simulink model "FloatShield_PID_Alternative"  (R2019a)
settings: Solver=FixedStepDiscrete  StartTime=0.0  StopTime=Inf  FixedStep=0.025  RelTol=1e-3
libraries: FloatLibrary x1, simulink x1
settings Model: SimulationMode=external  ExtModeTrigDuration=1  Creator=Peter  LastModifiedBy=Peter
settings OptimizationCC: EnhancedBackFolding=on  PassReuseOutputArgsAs=Individual arguments  MaxStackSize=64  OptimizeBlockOrder=speed  DifferentSizesBufferReuse=on  OptimizationCustomize=off
settings DebuggingCC: ParameterTunabilityLossMsg=error
settings HardwareCC: ProdBitPerInt=16  ProdBitPerPointer=16  ProdBitPerSizeT=16  ProdBitPerPtrDiffT=16  ProdLargestAtomicFloat=None  ProdWordSize=8  ProdHWDeviceType=Atmel->AVR
settings SFSimCC: MATLABDynamicMemAlloc=off
settings RTWCC: SystemTargetFile=ert.tlc  HardwareBoard=Arduino Uno  TLCOptions=-aInlineSetEventsForThisBaseRateFcn=TLC_FALSE -aSuppressMultiTaskScheduler=TLC_FALSE -aRateBasedStepFcn=1  TemplateMakefile=ert_default_tmf  GenerateReport=on  Toolchain=Arduino AVR  BuildConfiguration=Faster Runs  IncludeHyperlinkInReport=on  LaunchReport=on  GenerateTraceInfo=on  GenerateTraceReport=on  GenerateTraceReportSl=on  GenerateTraceReportSf=on  GenerateTraceReportEml=on
settings CodeAppCC: ForceParamTrailComments=on  IgnoreCustomStorageClasses=off  OperatorAnnotations=on  SimulinkDataObjDesc=on  SFDataObjDesc=on  InsertBlockDesc=on
settings ERTTargetCC: SupportContinuousTime=on  SupportVariableSizeSignals=on  ExtMode=on  ExtModeStaticAllocSize=250  ExtModeMexArgs='127.0.0.1' 0 17725

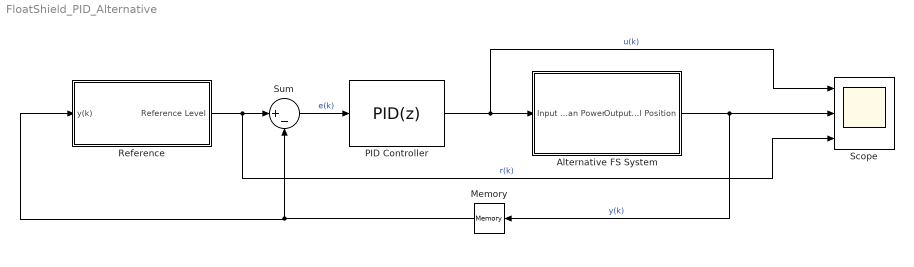
== system FloatShield_PID_Alternative ==
  Alternative FS System : Subsystem  mask{OutRadio=Percentage (%), Ncal=100, Ts=0.025}
      mask prompts: OutRadio "Output type"; Ncal "Calibration samples (-):"; Ts "Sampling period (s):"
      mask TypeOptions OutRadio: Percentage (%) | Altitude (mm)
      mask DialogControl DescGroupVar Prompt: FloatShield
      mask DialogControl DescTextVar Prompt: The block represents the FloatShield device. It accepts an input signal in the range of 0-100% that controls the fan power level and outputs ball position in form selected by the user. The block requires a sampling period and number of calibration samples out of which the extreme reading values will be computed using their mean value.
      mask Display: image('assets\FloatShield.svg');
  Memory : Memory  InheritSampleTime=on
  PID Controller : simulink/Continuous/PID Controller  Controller=PID  Form=Ideal  TimeDomain=Discrete-time  SampleTime=-1  IntegratorMethod=Forward Euler  FilterMethod=Forward Euler  ControllerParametersSource=internal  P=0.25  I=0.2  D=0.01  UseFilter=off  N=100  TunerSelectOption=Transfer Function Based (PID Tuner App)  InitialConditionSource=internal  InitialConditionForIntegrator=0  InitialConditionForFilter=0  DifferentiatorICPrevScaledInput=0  ExternalReset=none  TrackingMode=off  Kt=1  LimitOutput=on  UpperSaturationLimit=100  LowerSaturationLimit=30  LinearizeAsGain=on  AntiWindupMode=none  Kb=1  POutMin=[]  POutMax=[]  IOutMin=[]  IOutMax=[]  DOutMin=[]  DOutMax=[]  NOutMin=[]  NOutMax=[]  SumOutMin=[]  SumOutMax=[]  SaturationOutMin=[]  SaturationOutMax=[]  PParamMin=[]  PParamMax=[]  IParamMin=[]  IParamMax=[]  DParamMin=[]  DParamMax=[]  NParamMin=[]  NParamMax=[]  KbParamMin=[]  KbParamMax=[]  KtParamMin=[]  KtParamMax=[]  KbOutMin=[]  KbOutMax=[]  KtOutMin=[]  KtOutMax=[]  IntegratorOutMin=[]  IntegratorOutMax=[]  FilterOutMin=[]  FilterOutMax=[]  SumI1OutMin=[]  SumI1OutMax=[]  SumI2OutMin=[]  SumI2OutMax=[]  SumI3OutMin=[]  SumI3OutMax=[]  SumI4OutMin=[]  SumI4OutMax=[]  SumDOutMin=[]  SumDOutMax=[]  DifferentiatorOutMin=[]  DifferentiatorOutMax=[]  FilterDiffOutCoefMin=[]  FilterDiffOutCoefMax=[]  ReciprocalOutMin=[]  ReciprocalOutMax=[]  SumDenOutMin=[]  SumDenOutMax=[]  SumNumOutMin=[]  SumNumOutMax=[]  DivideOutMin=[]  DivideOutMax=[]  IntegratorContinuousStateAttributes=''  IntegratorStateMustResolveToSignalObject=off  IntegratorRTWStateStorageClass=Auto  FilterContinuousStateAttributes=''  FilterStateMustResolveToSignalObject=off  FilterRTWStateStorageClass=Auto  ParallelPVariant=Passthrough  IdealPVariant=InternalParameters  IVariant=InternalParameters  DVariant=InternalParameters  IntegratorVariant=Discrete  SatVariant=Enabled  AWVariant=Passthrough  PCopyVariant=Disabled  TRVariant=Disabled  FdbkBlocksVariant=Forward  IdealPFdbkVariant=Disabled  SatFdbkVariant=Disabled  DerivativeFilterVariant=Differentiator  NVariant=Passthrough  NCopyVariant=Disabled_SignalSpec  FilterICVariant=InternalICsDifferentiator  IntegratorICVariant=InternalICs  ExternalResetVariant=Disabled  TRSumVariant=Passthrough  SumFdbkVariant=Disabled  SumVariant=Sum_PID
  Reference : Subsystem  StopFcn=|  mask{RefVect=[65, 50, 35, 45, 60, 75, 55, 40, 20, 30], SectLen=2400, Ts=0.025}
      | if exist('simout')
      | structVar=simout;
      | end
      | 
      | if exist('ScopeData')
      | structVar=ScopeData;
      | end
      | 
      | if exist('structVar')
      | [u,y,r]=structVar.signals.values;
      | unmodifiedResponse=[r,y,u];
      | SimulinkPIDResponse=[r,y,u];
      | sectLen = str2num(get_param(strcat(gcs,'/Reference'),'SectLen'));
      | refVect = str2num(get_param(strcat(gcs,'/Reference'),'RefVect'));
      | refLen = length(refVect);
      | responseLen=length(SimulinkPIDResponse(:,1));
      | badSamples = responseLen-sectLen*refLen+1;
      | if badSamples>=1
      | SimulinkPIDResponse=SimulinkPIDResponse(badSamples:end,:);
      | end
      | clear sectLen refVect refLen responseLen badSamples structVar r y u;
      | save SimulinkPIDResponse SimulinkPIDResponse;
      | plotPIDResponse(SimulinkPIDResponse,100);
      | end
      mask prompts: RefVect "Reference Vector:"; SectLen "Section Length (Number of Samples):"; Ts "Sampling Period (s):"
      mask init:
      | NofSamples = str2num(get_param(strcat(gcs,'/Alternative FS System'),'Ncal'));
      | FSSampling = str2num(get_param(strcat(gcs,'/Alternative FS System'),'Ts'));
      | CalibTime = 2*NofSamples*FSSampling+2;
      | CalibTime = round(CalibTime/Ts)*Ts;
      mask DialogControl DescGroupVar Prompt: Reference Block
      mask DialogControl DescTextVar Prompt: Block used to provide changing reference levels during simulation.
  Scope : Scope  NumInputPorts=3
  Sum : Sum  Inputs=|+-
  wires:
  PID Controller/1 -> Scope/1, Alternative FS System/1(Input Fan Power)  "u(k)"
  Sum/1 -> PID Controller/1  "e(k)"
  Reference/1(Reference Level) -> Sum/1, Scope/3  "r(k)"
  Alternative FS System/1(Output Ball Position) -> Scope/2, Memory/1  "y(k)"
  Memory/1 -> Reference/1(y(k)), Sum/2

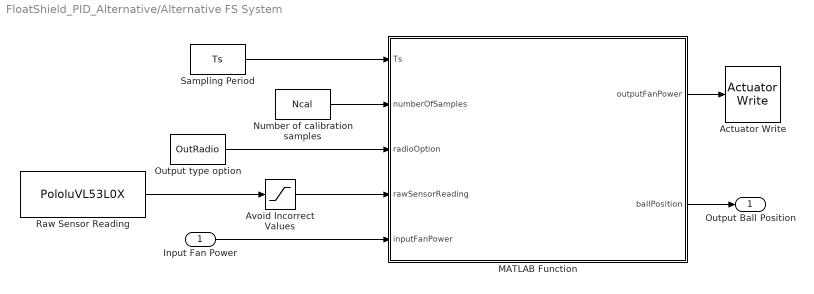
== system FloatShield_PID_Alternative/Alternative FS System ==
  Input Fan Power : Inport
  Actuator Write : FloatLibrary/Actuator Write
      settings: SourceProductName=AutomationShield
  Avoid Incorrect Values : Saturate  UpperLimit=345  LowerLimit=15
  MATLAB Function : MATLAB Function  TreatAsAtomicUnit=on
  Number of calibration samples : Constant  Value=Ncal  SampleTime=Ts
  Output type option : Constant  Value=OutRadio  SampleTime=Ts
  Raw Sensor Reading : S-Function  FunctionName=PololuVL53L0X  SFunctionModules='PololuVL53L0X_wrapper'  SFunctionDeploymentMode=off  EnableBusSupport=off
  Sampling Period : Constant  Value=Ts  SampleTime=Ts
  Output Ball Position : Outport
  wires:
  MATLAB Function/1(outputFanPower) -> Actuator Write/1
  Number of calibration samples/1 -> MATLAB Function/2(numberOfSamples)
  MATLAB Function/2(ballPosition) -> Output Ball Position/1
  Raw Sensor Reading/1 -> Avoid Incorrect Values/1
  Avoid Incorrect Values/1 -> MATLAB Function/4(rawSensorReading)
  Input Fan Power/1 -> MATLAB Function/5(inputFanPower)
  Sampling Period/1 -> MATLAB Function/1(Ts)
  Output type option/1 -> MATLAB Function/3(radioOption)

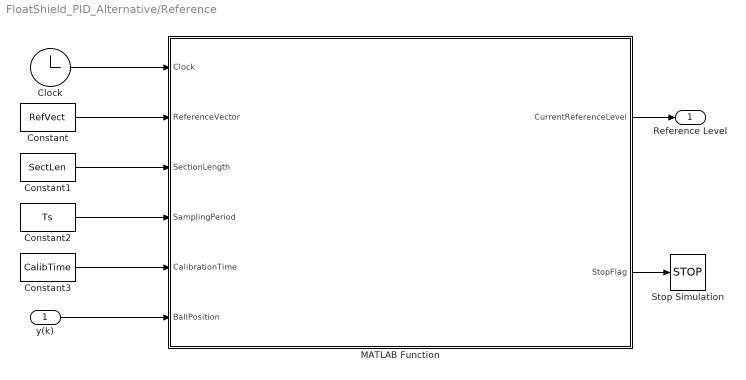
== system FloatShield_PID_Alternative/Reference ==
  y(k) : Inport
  Clock : Clock
  Constant : Constant  Value=RefVect  SampleTime=Ts
  Constant1 : Constant  Value=SectLen  SampleTime=Ts
  Constant2 : Constant  Value=Ts  SampleTime=Ts
  Constant3 : Constant  Value=CalibTime  SampleTime=Ts
  MATLAB Function : MATLAB Function  TreatAsAtomicUnit=on
  Stop Simulation : Stop
  Reference Level : Outport
  wires:
  Constant/1 -> MATLAB Function/2(ReferenceVector)
  Constant1/1 -> MATLAB Function/3(SectionLength)
  Constant2/1 -> MATLAB Function/4(SamplingPeriod)
  Clock/1 -> MATLAB Function/1(Clock)
  Constant3/1 -> MATLAB Function/5(CalibrationTime)
  MATLAB Function/1(CurrentReferenceLevel) -> Reference Level/1
  MATLAB Function/2(StopFlag) -> Stop Simulation/1
  y(k)/1 -> MATLAB Function/6(BallPosition)

== matlab function FloatShield_PID_Alternative/Alternative FS System/MATLAB Function ==
  data: Ts input; numberOfSamples input; radioOption input; rawSensorReading input; inputFanPower input; outputFanPower output; ballPosition output
%     Simulink Block representing FloatShield system.
%
%     This code is part of the AutomationShield hardware and software
%     ecosystem. Visit http://www.automationshield.com for more
%     details. This code is licensed under a Creative Commons
%     Attribution-NonCommercial 4.0 International License.
%
%     Created by Peter Chmurciak.
%     Last update: 13.8.2019.

function [outputFanPower, ballPosition] = fcn(Ts, numberOfSamples, radioOption, rawSensorReading, inputFanPower)

persistent iteration time calibrationStatus minVal maxVal;  % Persistent variables

if isempty(iteration)                                       % Initialisation
    iteration = 0;
    time = 0;
    calibrationStatus = 0;
    minVal = 0;
    maxVal = 0;
end

if calibrationStatus == 0                                  % Getting minimal value
    outputFanPower = 100;                                  % Set power output to max
    ballPosition = 0;
    if rawSensorReading < 100                              % Wait for ball to lift up
        time = time + Ts;
        if time >= 1                                       % Wait 1 second to stabilise
            iteration = iteration + 1;
            minVal = minVal + rawSensorReading;
            if iteration == numberOfSamples
                minVal = minVal / numberOfSamples;         % As average of N samples
                calibrationStatus = 1;
                time = 0;
                iteration = 0;
            end
        end
    end
elseif calibrationStatus == 1                              % Getting maximal value
    outputFanPower = 0;                                    % Set power output to zero
    ballPosition = 0;
    if rawSensorReading > 300                              % Wait for ball to fall
        time = time + Ts;
        if time >= 1                                       % Wait 1 second to stabilise
            iteration = iteration + 1;
            maxVal = maxVal + rawSensorReading;
            if iteration == numberOfSamples
                maxVal = maxVal / numberOfSamples;         % As average of N samples
                calibrationStatus = 2;
                time = 0;
                iteration = 0;
            end
        end
    end
else
    outputFanPower = inputFanPower;
    if radioOption == 1                                    % Output based on user choice
        ballPosition = constrain(map(rawSensorReading, maxVal, minVal, 0, 100), 0, 100);
    else
        ballPosition = constrain(map(rawSensorReading, maxVal, minVal, 0, maxVal-minVal), 0, maxVal);
    end
end

end                                                       % End of function definition

== matlab function FloatShield_PID_Alternative/Reference/MATLAB Function ==
  data: Clock input; CurrentReferenceLevel output; ReferenceVector input; SectionLength input; SamplingPeriod input; StopFlag output; CalibrationTime input; BallPosition input
%     Simulink Block for changing reference train used in PID examples.
%
%     This code is part of the AutomationShield hardware and software
%     ecosystem. Visit http://www.automationshield.com for more
%     details. This code is licensed under a Creative Commons
%     Attribution-NonCommercial 4.0 International License.
%
%     Created by Peter Chmurciak.
%     Last update: 12.8.2019.

function [CurrentReferenceLevel, StopFlag] = fcn(Clock, ReferenceVector, SectionLength, SamplingPeriod, CalibrationTime, BallPosition)

persistent counter liftTime;                            % Persistent variables

if Clock > CalibrationTime                              % Starts after calibration
    if isempty(liftTime)                                % Getting time when ball reaches half value of first reference level
        CurrentReferenceLevel = ReferenceVector(1);
        StopFlag = 0;
        if BallPosition > 0.5 * ReferenceVector(1)
            liftTime = Clock;
        end
    else                                                % Changing reference train
        if isempty(counter)
            counter = 1;
        end
        ReferenceLength = length(ReferenceVector);
        SectionDuration = SectionLength * SamplingPeriod;
        if (Clock - CalibrationTime - liftTime) <= (SectionDuration * counter)
            CurrentReferenceLevel = ReferenceVector(counter);
            StopFlag = 0;
        else
            counter = counter + 1;
            if counter <= ReferenceLength
                CurrentReferenceLevel = ReferenceVector(counter);
                StopFlag = 0;
            else
                CurrentReferenceLevel = ReferenceVector(counter-1);
                StopFlag = 1;                           % Stop simulation at the end of reference train
            end
        end
    end
else
    CurrentReferenceLevel = ReferenceVector(1);
    StopFlag = 0;
end

end                                                     % End of function definition
